simulink model "PID_lead_controllers_noise"  (R2023b)
settings: Solver=ode8  StartTime=0.0  StopTime=20  FixedStep=0.001  RelTol=1e-3
values from neighbouring files (symbols this model uses):
  K = p/z    [lead_vs_leadlag.m]    (also in setup_lead_controller.m)
  p = bodeoptions    [PID_lead_linmod.m]    (also in lead_vs_leadlag.m = 1/(alpha*T); setup_lead_controller.m = 1/(alpha*T))
  z = 1/T    [lead_vs_leadlag.m]    (also in setup_lead_controller.m)
settings Model: Creator=suvo  LastModifiedBy=suvo
settings SolverCC: AlgebraicLoopSolver=TrustRegion
settings DataIOCC: ReturnWorkspaceOutputs=off
settings DebuggingCC: UnconnectedInputMsg=warning  UnconnectedOutputMsg=warning  UnconnectedLineMsg=warning
settings ModelReferenceCC: EnableRefExpFcnMdlSchedulingChecks=on

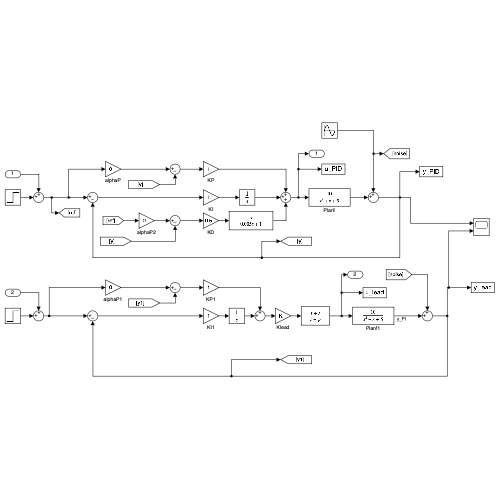
[thumbnail: Simulink's stored preview of the top-level diagram]
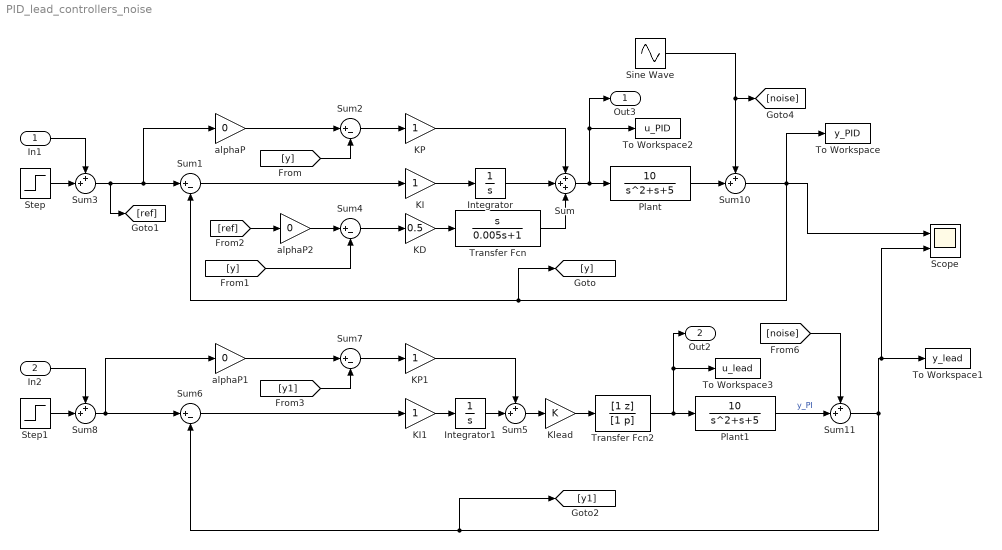
== system PID_lead_controllers_noise ==
  In1 : Inport
  In2 : Inport  Port=2
  Integrator : Integrator
  Integrator1 : Integrator
  KD : Gain  Gain=0.5
  KI : Gain
  KI1 : Gain
  KP : Gain
  KP1 : Gain
  Klead : Gain  Gain=K
  Plant : TransferFcn  Numerator=10  Denominator=[1 1 5]
  Plant1 : TransferFcn  Numerator=10  Denominator=[1 1 5]
  Scope : Scope  NumInputPorts=2
  Sine Wave : Sin  Amplitude=0.001  Frequency=50  SampleTime=0
  Step : Step  SampleTime=0
  Step1 : Step  SampleTime=0
  Sum : Sum  Inputs=+++
  Sum{1..2,4,6..7} (5 alike) : Sum  Inputs=|+-
  Sum{3,5,8,10..11} (5 alike) : Sum  Inputs=++|
  To Workspace : ToWorkspace  VariableName=y_PID  SaveFormat=Timeseries  SampleTime=-1
  To Workspace1 : ToWorkspace  VariableName=y_lead  SaveFormat=Timeseries  SampleTime=-1
  To Workspace2 : ToWorkspace  VariableName=u_PID  SaveFormat=Timeseries  SampleTime=-1
  To Workspace3 : ToWorkspace  VariableName=u_lead  SaveFormat=Timeseries  SampleTime=-1
  Transfer Fcn : TransferFcn  Numerator=[1 0]  Denominator=[0.005 1]
  Transfer Fcn2 : TransferFcn  Numerator=[1 z]  Denominator=[1 p]
  alphaP : Gain  Gain=0
  alphaP1 : Gain  Gain=0
  alphaP2 : Gain  Gain=0
  Out3 : Outport
  Out2 : Outport  Port=2
  wires:
  KI/1 -> Integrator/1
  Sum1/1 -> KI/1
  Sum3/1 -> alphaP/1, Sum1/1, [ref]
  Sum2/1 -> KP/1
  KP/1 -> Sum/1
  Integrator/1 -> Sum/2
  Sum/1 -> To Workspace2/1, Out3/1, Plant/1
  In1/1 -> Sum3/1
  Step/1 -> Sum3/2
  [y] -> Sum2/2
  KD/1 -> Transfer Fcn/1
  Transfer Fcn/1 -> Sum/3
  Sum4/1 -> KD/1
  [y] -> Sum4/2
  [ref] -> alphaP2/1
  alphaP/1 -> Sum2/1
  Sum6/1 -> KI1/1
  KP1/1 -> Sum5/1
  KI1/1 -> Integrator1/1
  In2/1 -> Sum8/1
  Sum7/1 -> KP1/1
  [y1] -> Sum7/2
  Integrator1/1 -> Sum5/2
  Sum8/1 -> alphaP1/1, Sum6/1
  Sum5/1 -> Klead/1
  alphaP1/1 -> Sum7/1
  Step1/1 -> Sum8/2
  Plant/1 -> Sum10/2
  Sum10/1 -> To Workspace/1, [y], Sum1/2, Scope/1
  Plant1/1 -> Sum11/2  "y_PI"
  Sum11/1 -> Scope/2, To Workspace1/1, [y1], Sum6/2
  [noise] -> Sum11/1
  Sine Wave/1 -> Sum10/1, [noise]
  Transfer Fcn2/1 -> Out2/1, To Workspace3/1, Plant1/1
  alphaP2/1 -> Sum4/1
  Klead/1 -> Transfer Fcn2/1
